simulink model "Single_Phase_Voltage_Amplitude"  (Simulink 7.5)
settings: Solver=ode15s  StartTime=0.0  StopTime=0.1  RelTol=1e-3
libraries: powerlib x8, powerlib_extras x3
settings Model: Creator=lm  LastModifiedBy=lm

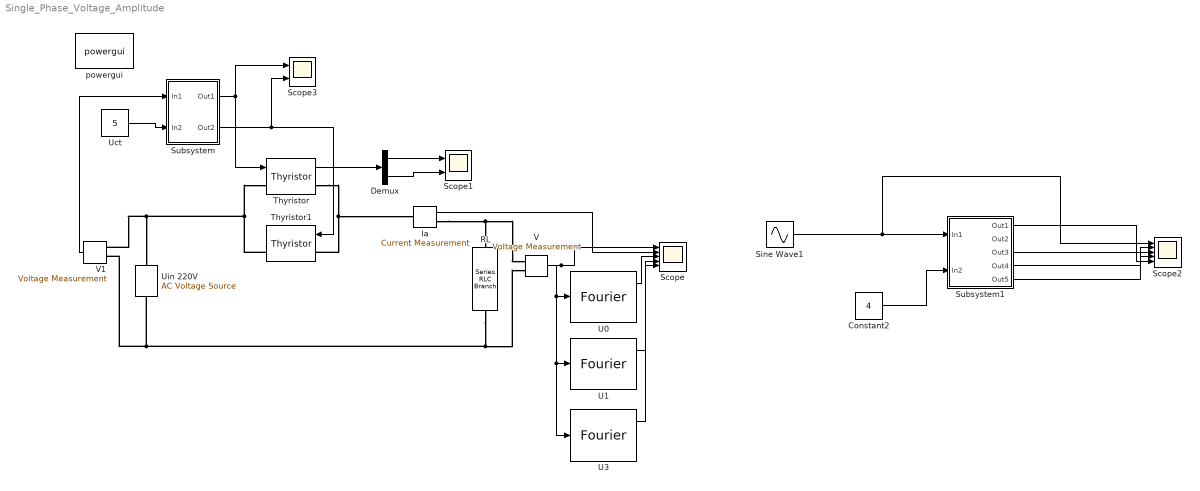
== system Single_Phase_Voltage_Amplitude ==
  Constant2 : Constant  Value=4  OutDataType=fixdt(1, 16)  OutScaling=2^0
  Demux : Demux  Outputs=2
  Ia : powerlib/Measurements/Current Measurement  DialogController=POWERSYS.PowerSysDialog  SystemSampleTime=-1  PhasorSimulation=off  OutputType=Complex  PSBequivalent=0
  RL : powerlib/Elements/Series RLC Branch  DialogController=POWERSYS.PowerSysDialog  PhysicalDomain=powersysdomain  SubClassName=unknown  LeftPortType=p1  RightPortType=p1  LConnTagsString=__new0  RConnTagsString=__new0  BranchType=RL  Resistance=1  Inductance=1e-2  SetiL0=off  InitialCurrent=0  Capacitance=1e-6  Setx0=off  InitialVoltage=0  Measurements=None
  Scope : Scope  NumInputPorts=5
      settings: YMin=-5~-5~-5~-5~-5  YMax=5~5~5~5~5
  Scope1 : Scope  NumInputPorts=2
      settings: YMin=-5~-5  YMax=5~5
  Scope2 : Scope  NumInputPorts=5
      settings: YMin=-5~-5~-5~-5~-5  YMax=5~5~5~5~5  SaveName=ScopeData2
  Scope3 : Scope  NumInputPorts=2
      settings: TimeRange=0.1  YMin=-5~-5  YMax=5~5  SaveName=ScopeData3
  Sine Wave1 : Sin  Amplitude=1  Bias=0  Frequency=100*pi  Phase=0  Samples=10  SampleTime=0  Offset=0
  Subsystem : Subsystem
  Subsystem1 : Subsystem
  Thyristor : powerlib/Power Electronics/Thyristor  DialogController=POWERSYS.PowerSysDialog  SystemSampleTime=-1  Ron=0.001  Lon=0  Vf=0.8  IC=0  Rs=500  Cs=250e-9  Measurements=on
  Thyristor1 : powerlib/Power Electronics/Thyristor  DialogController=POWERSYS.PowerSysDialog  SystemSampleTime=-1  Ron=0.001  Lon=0  Vf=0.8  IC=0  Rs=500  Cs=250e-9  Measurements=on
  U0 : powerlib_extras/Measurements/Fourier  DialogController=POWERSYS.PowerSysDialog  SystemSampleTime=-1  f1=50  n=0
  U1 : powerlib_extras/Measurements/Fourier  DialogController=POWERSYS.PowerSysDialog  SystemSampleTime=-1  f1=50  n=1
  U3 : powerlib_extras/Measurements/Fourier  DialogController=POWERSYS.PowerSysDialog  SystemSampleTime=-1  f1=50  n=3
  Uct : Constant  Value=5  OutDataType=fixdt(1, 16)  OutScaling=2^0
  Uin 220V : powerlib/Electrical Sources/AC Voltage Source  DialogController=POWERSYS.PowerSysDialog  SystemSampleTime=-1  Amplitude=220  Phase=0  Frequency=50  SampleTime=0  Measurements=None
  V : powerlib/Measurements/Voltage Measurement  DialogController=POWERSYS.PowerSysDialog  SystemSampleTime=-1  PhasorSimulation=off  OutputType=Complex  PSBequivalent=0
  V1 : powerlib/Measurements/Voltage Measurement  DialogController=POWERSYS.PowerSysDialog  SystemSampleTime=-1  PhasorSimulation=off  OutputType=Complex  PSBequivalent=0
  powergui : powerlib/powergui  Priority=1  SystemSampleTime=-1  SimulationMode=Discrete  SampleTime=50e-6  frequency=60  SPID=off  DisableSnubberDevices=off  DisableRonSwitches=off  DisableVfSwitches=off  SwTol=0  Interpol=off  frequencyindice=50  echomessages=off  HookPort=off  DisplayEquations=off  FunctionMessages=off  EnableUseOfTLC=off  x0status=blocks  RestoreLinks=warning  ResistiveCurrentMeasurement=off  Ylog=off  Xlog=on  ShowGrid=off  save=off  variable=ZData  ZoomFFT=off  StartTime=0.0  cycles=1  DisplayStyle=1  FreqAxis=off  MaxFrequency=1000  frequencyindicesteady=1  display=off  methode=off
  wires:
  V/1 -> Scope/1, U1/1, U3/1, U0/1
  Ia/1 -> Scope/2
  Uct/1 -> Subsystem/2(In2)
  Constant2/1 -> Subsystem1/2(In2)
  Sine Wave1/1 -> Scope2/1, Subsystem1/1(In1)
  Subsystem1/3(Out3) -> Scope2/2
  Subsystem1/4(Out4) -> Scope2/3
  Subsystem1/5(Out5) -> Scope2/4
  Subsystem1/1(Out1) -> Scope2/5
  V1/1 -> Subsystem/1(In1)
  Subsystem/1(Out1) -> Thyristor/1, Scope3/1
  Subsystem/2(Out2) -> Thyristor1/1, Scope3/2
  Thyristor/1 -> Demux/1
  Demux/1 -> Scope1/1
  Demux/2 -> Scope1/2
  U1/1 -> Scope/4
  U3/1 -> Scope/5
  U0/1 -> Scope/3
  connections:
  Thyristor1/RConn1 -- Thyristor/LConn1 -- Uin 220V/RConn1 -- V1/LConn1
  Thyristor/RConn1 -- Thyristor1/LConn1 -- Ia/LConn1
  Ia/RConn1 -- RL/LConn1 -- V/LConn1
  RL/RConn1 -- V/LConn2 -- Uin 220V/LConn1 -- V1/LConn2

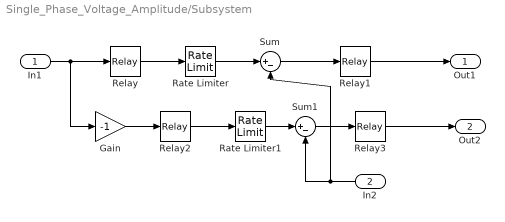
== system Single_Phase_Voltage_Amplitude/Subsystem ==
  In1 : Inport  OutDataType=fixdt(1, 16)  OutScaling=2^0
  In2 : Inport  Port=2  OutDataType=fixdt(1, 16)  OutScaling=2^0
  Gain : Gain  Gain=-1  ParameterDataType=fixdt(1, 16)  ParameterScaling=2^0  OutDataType=fixdt(1, 16)  OutScaling=2^0
  Rate Limiter : RateLimiter  RisingSlewLimit=1000  FallingSlewLimit=-1e8  SampleTimeMode=inherited
  Rate Limiter1 : RateLimiter  RisingSlewLimit=1000  FallingSlewLimit=-1e9  SampleTimeMode=inherited
  Relay : Relay  OnOutputValue=10  OutDataType=fixdt(1, 16)  OutScaling=2^0
  Relay1 : Relay  OutDataType=fixdt(1, 16)  OutScaling=2^0
  Relay2 : Relay  OnOutputValue=10  OutDataType=fixdt(1, 16)  OutScaling=2^0
  Relay3 : Relay  OutDataType=fixdt(1, 16)  OutScaling=2^0
  Sum : Sum  Inputs=|+-  OutDataType=fixdt(1, 16)  OutScaling=2^0
  Sum1 : Sum  Inputs=|+-  OutDataType=fixdt(1, 16)  OutScaling=2^0
  Out1 : Outport  OutDataType=fixdt(1, 16)  OutScaling=2^0
  Out2 : Outport  Port=2  OutDataType=fixdt(1, 16)  OutScaling=2^0
  wires:
  Relay1/1 -> Out1/1
  Sum/1 -> Relay1/1
  In1/1 -> Relay/1, Gain/1
  Gain/1 -> Relay2/1
  Relay2/1 -> Rate Limiter1/1
  Rate Limiter1/1 -> Sum1/1
  In2/1 -> Sum1/2, Sum/2
  Sum1/1 -> Relay3/1
  Relay3/1 -> Out2/1
  Relay/1 -> Rate Limiter/1
  Rate Limiter/1 -> Sum/1

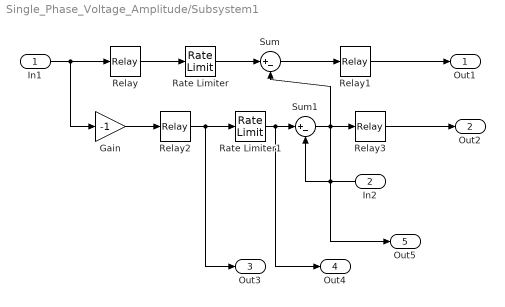
== system Single_Phase_Voltage_Amplitude/Subsystem1 ==
  In1 : Inport  OutDataType=fixdt(1, 16)  OutScaling=2^0
  In2 : Inport  Port=2  OutDataType=fixdt(1, 16)  OutScaling=2^0
  Gain : Gain  Gain=-1  ParameterDataType=fixdt(1, 16)  ParameterScaling=2^0  OutDataType=fixdt(1, 16)  OutScaling=2^0
  Rate Limiter : RateLimiter  RisingSlewLimit=1000  FallingSlewLimit=-1e8  SampleTimeMode=inherited
  Rate Limiter1 : RateLimiter  RisingSlewLimit=1000  FallingSlewLimit=-1e9  SampleTimeMode=inherited
  Relay : Relay  OnOutputValue=10  OutDataType=fixdt(1, 16)  OutScaling=2^0
  Relay1 : Relay  OutDataType=fixdt(1, 16)  OutScaling=2^0
  Relay2 : Relay  OnOutputValue=10  OutDataType=fixdt(1, 16)  OutScaling=2^0
  Relay3 : Relay  OutDataType=fixdt(1, 16)  OutScaling=2^0
  Sum : Sum  Inputs=|+-  OutDataType=fixdt(1, 16)  OutScaling=2^0
  Sum1 : Sum  Inputs=|+-  OutDataType=fixdt(1, 16)  OutScaling=2^0
  Out1 : Outport  OutDataType=fixdt(1, 16)  OutScaling=2^0
  Out2 : Outport  Port=2  OutDataType=fixdt(1, 16)  OutScaling=2^0
  Out3 : Outport  Port=3  OutDataType=fixdt(1, 16)  OutScaling=2^0
  Out4 : Outport  Port=4  OutDataType=fixdt(1, 16)  OutScaling=2^0
  Out5 : Outport  Port=5  OutDataType=fixdt(1, 16)  OutScaling=2^0
  wires:
  Rate Limiter/1 -> Sum/1
  Relay/1 -> Rate Limiter/1
  Relay3/1 -> Out2/1
  Sum1/1 -> Out5/1, Relay3/1
  In2/1 -> Sum/2, Sum1/2
  Rate Limiter1/1 -> Out4/1, Sum1/1
  Relay2/1 -> Out3/1, Rate Limiter1/1
  Gain/1 -> Relay2/1
  In1/1 -> Gain/1, Relay/1
  Sum/1 -> Relay1/1
  Relay1/1 -> Out1/1
